simulink model "sgMdl_IO3xx_CamCrank_Loopback"  (R2024b)
settings: Solver=FixedStepAuto  StartTime=0.0  StopTime=inf  RelTol=1e-3  EnableMultiTasking=on
undefined symbols (not defined in the file): Pull, pull, up
libraries: speedgoatlib_fpga_cam_crank x5, speedgoatlib_fpga x1
Description:
  | CamCrank_Loopback
settings Model: ModifiedByFormat=Speedgoat  SimulationMode=external  ExtModeTrigDuration=100000  Creator=Speedgoat  LastModifiedBy=Speedgoat
settings SolverCC: ConcurrentTasks=on  AlgebraicLoopSolver=TrustRegion  PositivePriorityOrder=on  AutoInsertRateTranBlk=on  InsertRTBMode=Never (minimum delay)
settings DataIOCC: SaveFormat=StructureWithTime
settings OptimizationCC: BlockReduction=off  OptimizeBlockIOStorage=off  BufferReuse=off  ReuseModelBlockBuffer=off
settings DebuggingCC: UnderspecifiedInitializationDetection=Classic  MergeDetectMultiDrivingBlocksExec=none  TasksWithSamePriorityMsg=none
settings HardwareCC: ProdBitPerLong=64  ProdLongLongMode=on  ProdHWDeviceType=Intel->x86-64 (Linux 64)
settings ModelReferenceCC: EnableRefExpFcnMdlSchedulingChecks=on  PropagateSignalLabelsOutOfModel=off
settings RTWCC: Description=Speedgoat Real-Time Target Machine  SystemTargetFile=speedgoat.tlc  TLCOptions=-axpcCPUClockPoll=0  TemplateMakefile=slrealtime_default_tmf  Toolchain=Simulink Real-Time Toolchain  BuildConfiguration=Faster Runs  TargetLang=C++  GPUComputeCapability=3.5  DLArmComputeVersion=19.05
settings SimulinkRealTimeTargetCC: SubcomponentCodeInterfacePackaging=Reusable function  InstructionSetFMA=off  LogToMDFFile=off  SLRTFileLogMaxRuns=10  UseGCCFastMath=on
settings ConfigComp: CovBoundaryAbsTol=1.0e-5

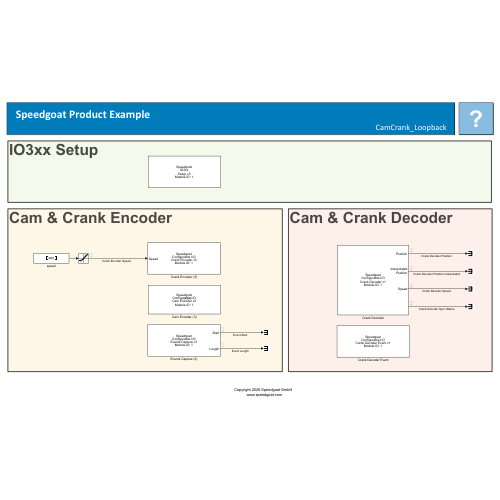
[thumbnail: Simulink's stored preview of the top-level diagram]
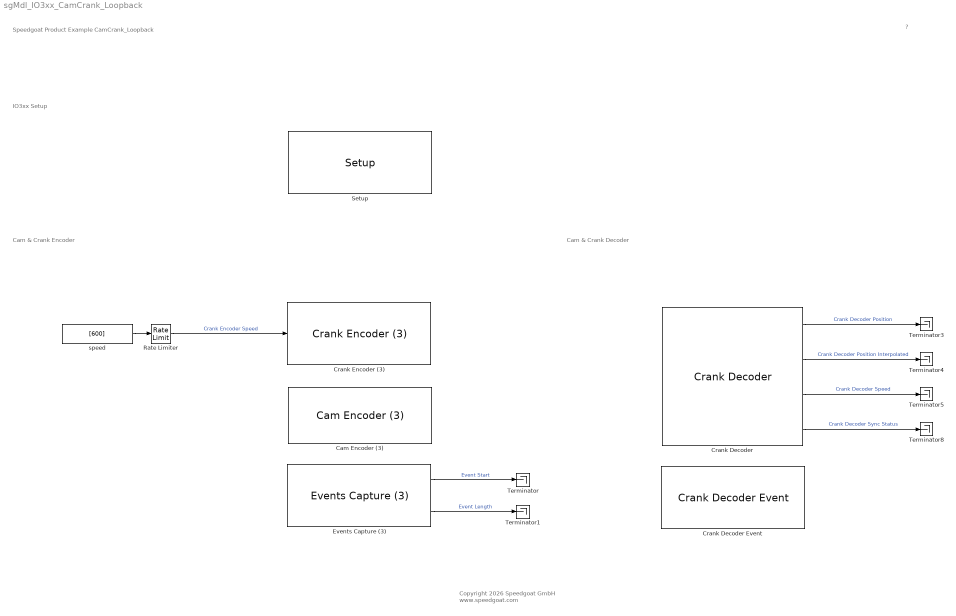
== system sgMdl_IO3xx_CamCrank_Loopback ==
  note: Cam & Crank Encoder
  note: IO3xx Setup
  note: Cam & Crank Decoder
  note: Speedgoat Product Example
      | CamCrank_Loopback
  note: ?
  note: Copyright 2026 Speedgoat GmbH
      |  www.speedgoat.com
  Cam Encoder (3) : speedgoatlib_fpga_cam_crank/Cam Encoder (3)  id=1  chan=[1]  ts=1e-3  initial_start=[[30,0,0,0,0,0,0,0,0,0]']  initial_length=[[90,0,0,0,0,0,0,0,0,0]']  show_start_and_length_input=off
      settings: SourceProductName=Simulink Real-Time: Speedgoat I/O Blockset
  Crank Decoder : speedgoatlib_fpga_cam_crank/Crank Decoder  id=1  chan=[1]  ts=1e-3  crankTeeth=60  crankTeethMissing=2  crankTeethMissingHigh=off  camToothOffset=[30]  camToothSize=[12]  TDCpulse=180  TDCpulseDuration=1e-3  startPulseDuration=1e-3  showRound=off  showPosition=on  showIntPosition=on  showSpeed=on  showSynch=on
      settings: SourceProductName=Simulink Real-Time: Speedgoat I/O Blockset
  Crank Decoder Event : speedgoatlib_fpga_cam_crank/Crank Decoder Event  id=1  chan=[1]  ts=1e-3  eventPulse=[90]  eventPulseDuration=[1e-3]  crankMaster=1  crankTeeth=60  crankTeethMissing=2
      settings: SourceProductName=Simulink Real-Time: Speedgoat I/O Blockset
  Crank Encoder (3) : speedgoatlib_fpga_cam_crank/Crank Encoder (3)  id=1  chan=[1]  ts=1e-3  start_angle=[0]  speed=0  number_of_crank_teeth=60  number_of_missing_crank_teeth=2  duty_cycle=0.5  invert_crankshaft=off  tdc_start=0.0  tdc_length=0.0  show_speed_input=on  show_duty_cycle_input=off  show_position_output=off
      settings: SourceProductName=Simulink Real-Time: Speedgoat I/O Blockset
  Events Capture (3) : speedgoatlib_fpga_cam_crank/Events Capture (3)  id=1  crank_channel=[1]  chan=[1]  ts=1e-3  debounce=100e-9  debounce_eff=106.7e-9  events_width=1  show_start=on  show_length=on
      settings: SourceProductName=Simulink Real-Time: Speedgoat I/O Blockset
  Rate Limiter : RateLimiter  RisingSlewLimit=600  FallingSlewLimit=-600  SampleTimeMode=inherited
  Setup : speedgoatlib_fpga/Setup/Setup  board=Please select...  id=1  pciSlot=-1  device_id=1  bitstreamFilePath=[]  bitstreamFile=<Manual entry>  fpgaFreq=73.73 MHz  enableDma=off  rearEnb_1=off  rearIO_1=None  rearEnb_2=off  rearIO_2=None  ProgSpiFlash=off  ProgBPIFlash=off  useFpgaDmaController=off  dmaTrigDropdown=Model Step  dmaTrigSelect=0  dmaStopOnOverload=on  dmaModeSequential=on  dmaModeParallel=off  PullRPort15=pull-up 3.3V  PullRPort31=pull-up 3.3V  PullRPort47=pull-up 3.3V  PullRPort63=pull-up 3.3V  diffLineTermination_1=on  diffLineTermination_2=on  diffLineTermination_3=on  diffLineTermination_4=on  diffLineTermination_5=on  diffLineTermination_6=on  diffLineTermination_7=on  diffLineTermination_8=on  diffLineTermination_9=on  diffLineTermination_10=on  diffLineTermination_11=on  diffLineTermination_12=on  diffLineTermination_13=on  diffLineTermination_14=on  diffLineTermination_15=on  diffLineTermination_16=on  diffLineTermination_17=on  diffLineTermination_18=on  diffLineTermination_19=on  diffLineTermination_20=on  diffLineTermination_21=on  diffLineTermination_22=on  diffLineTermination_23=on  diffLineTermination_24=on  diffLineTermination_25=on  diffLineTermination_26=on  diffLineTermination_27=on  diffLineTermination_28=on  diffLineTermination_29=on  diffLineTermination_30=on  diffLineTermination_31=on  diffLineTermination_32=on  ioVoltageDropDown1=3.3V  pullResistorDropDown1_1=Pull-up  pullResistorDropDown1_2=Pull-up  pullResistorDropDown1_3=Pull-up  pullResistorDropDown1_4=Pull-up  pullResistorDropDown1_5=Pull-up  pullResistorDropDown1_6=Pull-up  pullResistorDropDown1_7=Pull-up  pullResistorDropDown1_8=Pull-up  ttlIsImplementedCheckBox1=off  pullResistorDropDown2=Pull-up  ioVoltageDropDown2=3.3V  ttlIsImplementedCheckBox2=off  pullResistorDropDown3=Pull-up  ioVoltageDropDown3=3.3V  ttlIsImplementedCheckBox3=off  pullResistorDropDown4=Pull-up  ioVoltageDropDown4=3.3V  ttlIsImplementedCheckBox4=off  pullResistorDropDown5=Pull-up  ioVoltageDropDown5=3.3V  ttlIsImplementedCheckBox5=off  pullResistorDropDown6=Pull-up  ioVoltageDropDown6=3.3V  ttlIsImplementedCheckBox6=off  pullResistorDropDown7=Pull-up  ioVoltageDropDown7=3.3V  ttlIsImplementedCheckBox7=off  pullResistorDropDown8=Pull-up  ioVoltageDropDown8=3.3V  ttlIsImplementedCheckBox8=off  terminationCheckBox1=off  terminationCheckBox2=off  terminationCheckBox3=off  terminationCheckBox4=off  diffIsImplementedCheckBox1=off  terminationCheckBox5=off  terminationCheckBox6=off  terminationCheckBox7=off  terminationCheckBox8=off  diffIsImplementedCheckBox2=off  terminationCheckBox9=off  terminationCheckBox10=off  terminationCheckBox11=off  terminationCheckBox12=off  diffIsImplementedCheckBox3=off  terminationCheckBox13=off  terminationCheckBox14=off  terminationCheckBox15=off  terminationCheckBox16=off  diffIsImplementedCheckBox4=off  terminationCheckBox17=off  terminationCheckBox18=off  terminationCheckBox19=off  terminationCheckBox20=off  diffIsImplementedCheckBox5=off  terminationCheckBox21=off  terminationCheckBox22=off  terminationCheckBox23=off  terminationCheckBox24=off  diffIsImplementedCheckBox6=off  terminationCheckBox25=off  terminationCheckBox26=off  terminationCheckBox27=off  terminationCheckBox28=off  diffIsImplementedCheckBox7=off  terminationCheckBox29=off  terminationCheckBox30=off  terminationCheckBox31=off  terminationCheckBox32=off  diffIsImplementedCheckBox8=off  PullRPort0_1=pull-up  VioPort0_1=3.3V  PullRPort1_1=pull-up  VioPort1_1=3.3V  PullRPort2_1=pull-up  VioPort2_1=3.3V  PullRPort3_1=pull-up  VioPort3_1=3.3V  PullRPort4_1=pull-up  VioPort4_1=3.3V  PullRPort5_1=pull-up  VioPort5_1=3.3V  PullRPort6_1=pull-up  VioPort6_1=3.3V  diffLineTermination_rear1_1=on  diffLineTermination_rear1_2=on  diffLineTermination_rear1_3=on  diffLineTermination_rear1_4=on  diffLineTermination_rear1_5=on  diffLineTermination_rear1_6=on  diffLineTermination_rear1_7=on  diffLineTermination_rear1_8=on  PullRPort0_2=pull-up  VioPort0_2=3.3V  PullRPort1_2=pull-up  VioPort1_2=3.3V  PullRPort2_2=pull-up  VioPort2_2=3.3V  PullRPort3_2=pull-up  VioPort3_2=3.3V  PullRPort4_2=pull-up  VioPort4_2=3.3V  PullRPort5_2=pull-up  VioPort5_2=3.3V  PullRPort6_2=pull-up  VioPort6_2=3.3V  diffLineTermination_rear2_1=on  diffLineTermination_rear2_2=on  diffLineTermination_rear2_3=on  diffLineTermination_rear2_4=on  diffLineTermination_rear2_5=on  diffLineTermination_rear2_6=on  diffLineTermination_rear2_7=on  diffLineTermination_rear2_8=on
      settings: SourceProductName=Simulink Real-Time: Speedgoat I/O Blockset
  Terminator{,1,3..5,8} (6 alike) : Terminator
  speed : Constant  Value=[600]  SampleTime=-1
  wires:
  speed/1 -> Rate Limiter/1
  Rate Limiter/1 -> Crank Encoder (3)/1  "Crank Encoder Speed"
  Events Capture (3)/1 -> Terminator/1  "Event Start"
  Events Capture (3)/2 -> Terminator1/1  "Event Length"
  Crank Decoder/3 -> Terminator5/1  "Crank Decoder Speed"
  Crank Decoder/2 -> Terminator4/1  "Crank Decoder Position Interpolated"
  Crank Decoder/1 -> Terminator3/1  "Crank Decoder Position"
  Crank Decoder/4 -> Terminator8/1  "Crank Decoder Sync Status"
